simulink model "untitled2"  (R2023a)
settings: Solver=FixedStepAuto  StartTime=0.0  StopTime=4  FixedStep=1e-5  RelTol=1e-3
undefined symbols (not defined in the file): IaN, J, Ka, Kav, Ki, Kiv, Kp, Kpv, KT, La, Ra, Tfi, Tfv, UaN
libraries: spsMosfetLib x16, spsDCMachineLib x4, spsDCVoltageSourceLib x4, simulink x4, spsVoltageMeasurementLib x4, sps_lib x1
settings Model: Creator=luand  LastModifiedBy=luand

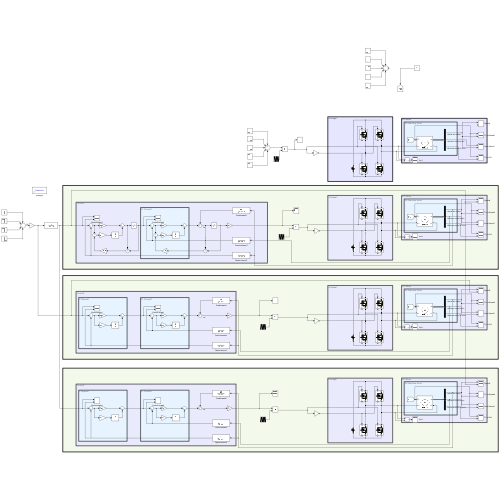
[thumbnail: Simulink's stored preview of the top-level diagram]
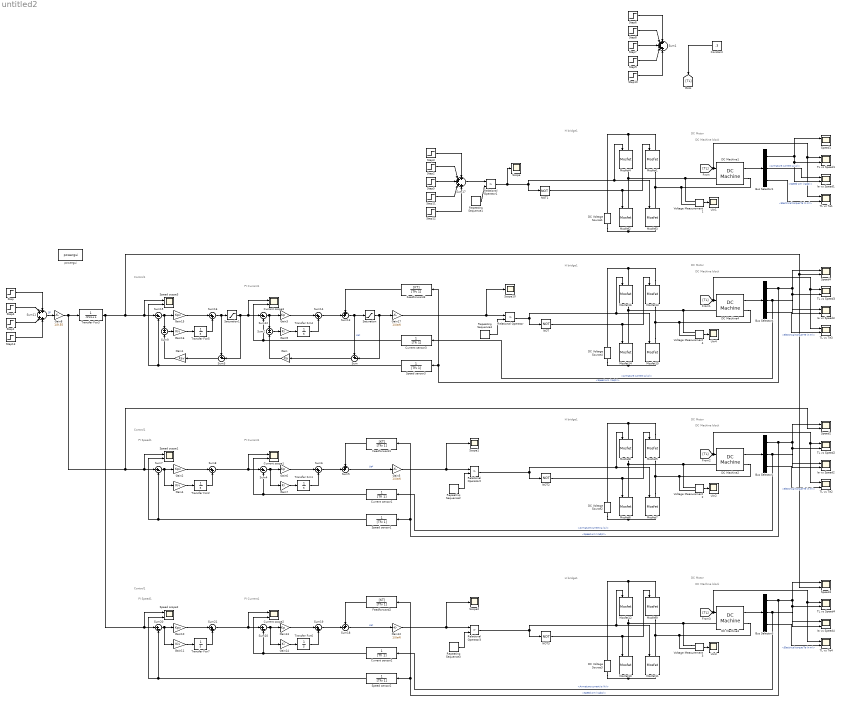
== system untitled2 ==
  note: PI Current1
  note: Control1
  note: H bridge1
  note: DC Motor
  note: DC Machine block
  note: H bridge1
  note: DC Motor
  note: DC Machine block
  note: PI Current1
  note: Control1
  note: H bridge1
  note: DC Motor
  note: DC Machine block
  note: PI Speed1
  note: PI Current1
  note: Control1
  note: H bridge1
  note: DC Motor
  note: DC Machine block
  note: PI Speed1
  Bus Selector{1..4} (4 alike) : BusSelector  OutputSignals=Speed wm (rad/s),Armature current ia (A),Electrical torque Te (n m)
  Constant : Constant  Value=.3
  Current scope1 : Scope  NumInputPorts=2
  Current scope2 : Scope  NumInputPorts=2
  Current scope3 : Scope  NumInputPorts=2
  Current sensor1 : TransferFcn  Denominator=[Tfi 1]
  Current sensor2 : TransferFcn  Denominator=[Tfi 1]
  Current sensor3 : TransferFcn  Denominator=[Tfi 1]
  DC Machine{1..4} (4 alike) : spsDCMachineLib/DC Machine  PresetModel=No  MechanicalLoad=Torque TL  FieldType=Permanent magnet  ShowDetailedParameters=on  MeasurementBus=off  RLa=[ Ra La ]  RLf="[ 240  120]"  Laf=1.8  MachineConstant=Torque constant (N.m/A)  Ke=1.8  Kt=KT  J=J  Bm=0  Tf=0  w0=0  Ifinit=1  TsPowergui=0  TsBlock=-1
  DC Voltage Source{1..4} (4 alike) : spsDCVoltageSourceLib/DC Voltage Source  Amplitude=UaN  Measurements=None
  Feedforward1 : TransferFcn  Numerator=[KT]  Denominator=[Tfv 1]
  Feedforward2 : TransferFcn  Numerator=[KT]  Denominator=[Tfv 1]
  Feedforward3 : TransferFcn  Numerator=[KT]  Denominator=[Tfv 1]
  Gain : Gain  Gain=Ka
  Gain1 : Gain  Gain=Kav
  Gain10 : Gain  Gain=Kpv
  Gain11 : Gain  Gain=Kiv
  Gain12 : Gain  Gain=1/UaN
  Gain13 : Gain  Gain=Kp
  Gain14 : Gain  Gain=Ki
  Gain15 : Gain  Gain=Kpv
  Gain16 : Gain  Gain=Kiv
  Gain17 : Gain  Gain=1/UaN
  Gain2 : Gain  Gain=Kpv
  Gain3 : Gain  Gain=Kp
  Gain4 : Gain  Gain=Kiv
  Gain5 : Gain  Gain=1/UaN
  Gain6 : Gain  Gain=Kp
  Gain7 : Gain  Gain=Ki
  Gain8 : Gain  Gain=1/9.55
  Gain9 : Gain  Gain=Ki
  Ia vs Speed{1..4} (4 alike) : Scope  NumInputPorts=2
  Mosfet{1..16} (16 alike) : spsMosfetLib/Mosfet  Ron=1e-3  Lon=0  Rd=0.01  Vfd=0  IC=0  Rs=1e5  Cs=inf  Measurements=on
  NOT{,1..3} (4 alike) : Logic  Operator=NOT  IconShape=distinctive  AllPortsSameDT=off  OutDataTypeStr=boolean
  Relational Operator{,1..3} (4 alike) : RelationalOperator  Operator=>  OutDataTypeStr=boolean  RndMeth=Simplest  InputSameDT=off
  Repeating Sequence{1..4} (4 alike) : simulink/Sources/Repeating Sequence  rep_seq_t=[0 5e-4 1e-3]  rep_seq_y=[-1 1 -1]
  Saturation : Saturate  UpperLimit=UaN  LowerLimit=-UaN
  Saturation1 : Saturate  UpperLimit=7*IaN  LowerLimit=-7*IaN
  Scope{,1..2,10} (4 alike) : Scope
  Speed scope1 : Scope  NumInputPorts=2
  Speed scope2 : Scope  NumInputPorts=2
  Speed scope3 : Scope  NumInputPorts=2
  Speed sensor1 : TransferFcn  Denominator=[Tfv 1]
  Speed sensor2 : TransferFcn  Denominator=[Tfv 1]
  Speed sensor3 : TransferFcn  Denominator=[Tfv 1]
  Speed{1..4} (4 alike) : Scope  NumInputPorts=2
  Step : Step  Time=0  After=3000  SampleTime=0
  Step1 : Step  Time=2  After=-3000  SampleTime=0
  Step10 : Step  Time=2.5  After=5  SampleTime=0
  Step11 : Step  Time=0  After=-.4  SampleTime=0
  Step12 : Step  Time=0  After=-.6  SampleTime=0
  Step13 : Step  Time=3  After=-1000  SampleTime=0
  Step2 : Step  After=-.4  SampleTime=0
  Step3 : Step  Time=0  SampleTime=0
  Step4 : Step  After=-2000  SampleTime=0
  Step5 : Step  Time=0  After=-.6  SampleTime=0
  Step6 : Step  Time=.5  After=5  SampleTime=0
  Step7 : Step  Time=1.5  After=5  SampleTime=0
  Step8 : Step  After=-5  SampleTime=0
  Step9 : Step  Time=2  After=-5  SampleTime=0
  Sum : Sum  Inputs=+-|
  Sum1 : Sum  Inputs=+++++
  Sum{4,7,10,12,15,20} (6 alike) : Sum  Inputs=|+-
  Sum11 : Sum  Inputs=++|++
  Sum13 : Sum  Inputs=++|
  Sum{6,8,14,16,19,21} (6 alike) : Sum  Inputs=|++
  Sum17 : Sum  Inputs=+++++
  Sum18 : Sum  Inputs=++|
  Sum2 : Sum  Inputs=+|-
  Sum3 : Sum  Inputs=+-|
  Sum5 : Sum  Inputs=++|
  Sum9 : Sum  Inputs=+|-
  TL vs Speed{1..4} (4 alike) : Scope  NumInputPorts=2
  TL vs Te{1..4} (4 alike) : Scope  NumInputPorts=2
  Transfer Fcn{1..2,4..7} (6 alike) : TransferFcn  Denominator=[1 0]
  Transfer Fcn3 : TransferFcn  Denominator=[.05 1]
  Uin{1..4} (4 alike) : Scope
  Voltage Measurement{1..4} (4 alike) : spsVoltageMeasurementLib/Voltage Measurement  PhasorSimulation=off  OutputType=Complex  PSBequivalent=0
  powergui : sps_lib/powergui  Priority=1  SimulationMode=Continuous  SampleTime=1e-5  frequency=60  Iterations=50  frequencyindice=0  Pbase=100e6  ErrMax=1e-4  UnitsV=kV  UnitsW=MW  buscounter=0  FunctionMessages=off  echomessages=off  EnableUseOfTLC=off  CurrentSourceSwitches=off  DisableSnubberDevices=off  DisableRonSwitches=off  DisableVfSwitches=off  DisplayEquations=off  AutomaticDiscreteSolvers=off  SolverType=Tustin/Backward Euler (TBE)  Interpol=off  ExternalGateDelay=off  methode=off  Ts=100  x0status=blocks  SPID=on  SwTol=0  HookPort=off  NonlinearTolerance=1e-4  nMaxIteration=100  ContinueOnMaxIteration=off  RestoreLinks=warning  ResistiveCurrentMeasurement=off  Frange=[0:2:500]  Ylog=off  Xlog=on  ShowGrid=off  save=off  variable=ZData  structure=0  ZoomFFT=off  StartTime=0.0  cycles=1  DisplayStyle=1  fundamental=60  FreqAxis=off  MaxFrequency=1000  frequencyindicesteady=1  RmsSteady=1  display=off
  wires:
  Bus Selector4/3 -> TL vs Te3/2  "<Electrical torque Te (n m)>"
  Repeating Sequence4/1 -> Relational Operator/2
  Transfer Fcn5/1 -> Sum16/2
  Voltage Measurement4/1 -> Uin4/1
  Gain3/1 -> Sum14/1
  Bus Selector4/2 -> Ia vs Speed3/1, Current sensor3/1  "<Armature current ia (A)>"
  Speed sensor3/1 -> Speed scope3/2, Sum15/2
  Gain9/1 -> Transfer Fcn4/1
  NOT/1 -> Mosfet14/1, Mosfet13/1
  Gain15/1 -> Sum16/1
  Sum13/1 -> Saturation/1, Sum/1  "Ua*"
  Sum15/1 -> Gain15/1, Sum9/1
  Sum12/1 -> Gain3/1, Sum2/1
  Gain16/1 -> Transfer Fcn5/1
  Transfer Fcn4/1 -> Sum14/2
  Sum14/1 -> Sum13/2
  Bus Selector4/1 -> Speed sensor3/1, Feedforward3/1, Ia vs Speed3/2, TL vs Speed3/2, Speed4/1  "<Speed wm (rad/s)>"
  DC Machine4/1 -> Bus Selector4/1
  Feedforward3/1 -> Sum13/1
  Current sensor3/1 -> Current scope3/2, Sum12/2
  Relational Operator/1 -> NOT/1, Mosfet15/1, Mosfet16/1
  Step1/1 -> Sum11/3
  Step/1 -> Sum11/1
  Sum11/1 -> Gain8/1  "SP"
  Step4/1 -> Sum11/2
  Step3/1 -> Sum17/1
  Step2/1 -> Sum17/2
  DC Machine1/1 -> Bus Selector1/1
  Voltage Measurement1/1 -> Uin1/1
  Gain17/1 -> Relational Operator/1, Scope10/1
  NOT1/1 -> Mosfet2/1, Mosfet1/1
  Relational Operator1/1 -> Scope/1, Mosfet3/1, Mosfet4/1, NOT1/1
  Bus Selector1/1 -> Speed1/1, TL vs Speed1/2, Ia vs Speed1/2  "<Speed wm (rad/s)>"
  Repeating Sequence1/1 -> Relational Operator1/2
  Sum17/1 -> Relational Operator1/1
  Step8/1 -> Sum1/2
  Step6/1 -> Sum1/1
  Step7/1 -> Sum1/3
  Step9/1 -> Sum1/4
  Step10/1 -> Sum1/5
  Saturation/1 -> Sum/2, Gain17/1
  Sum/1 -> Gain/1
  Gain/1 -> Sum2/2
  Sum2/1 -> Gain9/1
  Sum16/1 -> Sum3/1, Saturation1/1
  Sum8/1 -> Sum4/1, Current scope1/1
  Gain5/1 -> Scope1/1, Relational Operator2/1
  Relational Operator2/1 -> Mosfet8/1, Mosfet7/1, NOT2/1
  Current sensor1/1 -> Sum4/2, Current scope1/2
  Feedforward1/1 -> Sum5/1
  DC Machine2/1 -> Bus Selector2/1
  Bus Selector2/1 -> Speed2/1, TL vs Speed2/2, Ia vs Speed2/2, Speed sensor1/1, Feedforward1/1  "<Speed wm (rad/s)>"
  Sum6/1 -> Sum5/2
  Transfer Fcn1/1 -> Sum6/2
  Gain4/1 -> Transfer Fcn2/1
  Sum4/1 -> Gain7/1, Gain6/1
  Sum7/1 -> Gain2/1, Gain4/1
  Gain2/1 -> Sum8/1
  NOT2/1 -> Mosfet5/1, Mosfet6/1
  Gain7/1 -> Transfer Fcn1/1
  Speed sensor1/1 -> Sum7/2, Speed scope1/2
  Gain8/1 -> Transfer Fcn3/1, Sum7/1, Speed scope1/1, Speed2/2
  Bus Selector2/2 -> Current sensor1/1, Ia vs Speed2/1  "<Armature current ia (A)>"
  Gain6/1 -> Sum6/1
  Voltage Measurement2/1 -> Uin2/1
  Transfer Fcn2/1 -> Sum8/2
  Repeating Sequence2/1 -> Relational Operator2/2
  Bus Selector2/3 -> TL vs Te2/2  "<Electrical torque Te (n m)>"
  Sum5/1 -> Gain5/1  "Ua*"
  Saturation1/1 -> Sum3/2, Current scope3/1, Sum12/1
  Sum3/1 -> Gain1/1
  Gain1/1 -> Sum9/2
  Sum9/1 -> Gain16/1
  Transfer Fcn3/1 -> Speed scope2/1, Sum20/1, Speed4/2, Speed3/2, Speed scope3/1, Sum15/1
  Sum18/1 -> Gain12/1  "Ua*"
  Bus Selector3/3 -> TL vs Te4/2  "<Electrical torque Te (n m)>"
  Repeating Sequence3/1 -> Relational Operator3/2
  Transfer Fcn7/1 -> Sum21/2
  Voltage Measurement3/1 -> Uin3/1
  Gain13/1 -> Sum19/1
  Bus Selector3/2 -> Ia vs Speed4/1, Current sensor2/1  "<Armature current ia (A)>"
  Speed sensor2/1 -> Speed scope2/2, Sum20/2
  Gain14/1 -> Transfer Fcn6/1
  NOT3/1 -> Mosfet10/1, Mosfet9/1
  Gain10/1 -> Sum21/1
  Sum20/1 -> Gain11/1, Gain10/1
  Sum10/1 -> Gain13/1, Gain14/1
  Gain11/1 -> Transfer Fcn7/1
  Transfer Fcn6/1 -> Sum19/2
  Sum19/1 -> Sum18/2
  Bus Selector3/1 -> Feedforward2/1, Speed sensor2/1, Ia vs Speed4/2, TL vs Speed4/2, Speed3/1  "<Speed wm (rad/s)>"
  DC Machine3/1 -> Bus Selector3/1
  Feedforward2/1 -> Sum18/1
  Current sensor2/1 -> Current scope2/2, Sum10/2
  Relational Operator3/1 -> NOT3/1, Mosfet11/1, Mosfet12/1
  Gain12/1 -> Relational Operator3/1, Scope2/1
  Sum21/1 -> Current scope2/1, Sum10/1
  [TL] -> TL vs Te1/1, TL vs Speed1/1, DC Machine1/1
  [TL] -> TL vs Te3/1, TL vs Speed3/1, DC Machine4/1
  [TL] -> TL vs Te4/1, TL vs Speed4/1, DC Machine3/1
  Step5/1 -> Sum17/3
  Step11/1 -> Sum17/4
  Step12/1 -> Sum17/5
  [TL] -> TL vs Te2/1, TL vs Speed2/1, DC Machine2/1
  Bus Selector1/2 -> Ia vs Speed1/1  "<Armature current ia (A)>"
  Bus Selector1/3 -> TL vs Te1/2  "<Electrical torque Te (n m)>"
  Step13/1 -> Sum11/4
  Constant/1 -> [TL]
  connections:
  Mosfet15/LConn1 -- Voltage Measurement4/LConn2 -- DC Machine4/RConn1 -- Mosfet13/RConn1
  Mosfet13/LConn1 -- Mosfet16/LConn1 -- DC Voltage Source4/RConn1
  Mosfet15/RConn1 -- Mosfet14/RConn1 -- DC Voltage Source4/LConn1
  Mosfet4/LConn1 -- Mosfet1/LConn1 -- DC Voltage Source1/RConn1
  Mosfet2/RConn1 -- Mosfet3/RConn1 -- DC Voltage Source1/LConn1
  DC Machine1/LConn1 -- Voltage Measurement1/LConn1 -- Mosfet2/LConn1 -- Mosfet4/RConn1
  Mosfet1/RConn1 -- Voltage Measurement1/LConn2 -- DC Machine1/RConn1 -- Mosfet3/LConn1
  Mosfet7/LConn1 -- Mosfet5/RConn1 -- DC Machine2/RConn1 -- Voltage Measurement2/LConn2
  Mosfet5/LConn1 -- DC Voltage Source2/RConn1 -- Mosfet8/LConn1
  Mosfet7/RConn1 -- DC Voltage Source2/LConn1 -- Mosfet6/RConn1
  Mosfet8/RConn1 -- Voltage Measurement2/LConn1 -- DC Machine2/LConn1 -- Mosfet6/LConn1
  Mosfet16/RConn1 -- Mosfet14/LConn1 -- DC Machine4/LConn1 -- Voltage Measurement4/LConn1
  DC Machine3/RConn1 -- Mosfet11/LConn1 -- Mosfet9/RConn1 -- Voltage Measurement3/LConn2
  DC Voltage Source3/RConn1 -- Mosfet9/LConn1 -- Mosfet12/LConn1
  DC Voltage Source3/LConn1 -- Mosfet11/RConn1 -- Mosfet10/RConn1
  Voltage Measurement3/LConn1 -- Mosfet12/RConn1 -- Mosfet10/LConn1 -- DC Machine3/LConn1
